simulink model "Simulink_model"  (R2024b)
settings: Solver=FixedStepAuto  StartTime=0.0  StopTime=10.0  FixedStep=1e-3  RelTol=1e-3
values from neighbouring files (symbols this model uses):
  A = [0 1; 0 -10]    [Script.m]
  B = [0; 120]    [Script.m]
  C = [1 0]    [Script.m]
  D = 0    [Script.m]
  Kd = (2*delta*omega_n+(-lambda3)-10)/(120)    [Script.m]
  Ki = (omega_n^2*(-lambda3))/(120)    (= 36)    [Script.m]
  Kp = (omega_n^2+2*delta*omega_n*(-lambda3))/(120)    [Script.m]
  Tl = 1/(8 * omega_n)    (= 0.0104166666667)    [Script.m]
settings Model: Creator=andre  LastModifiedBy=Enrico 2

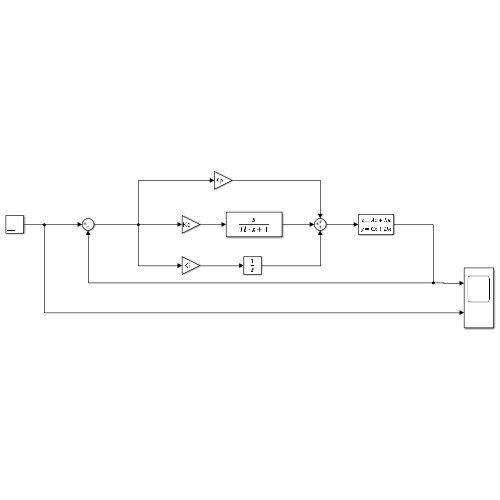
[thumbnail: Simulink's stored preview of the top-level diagram]
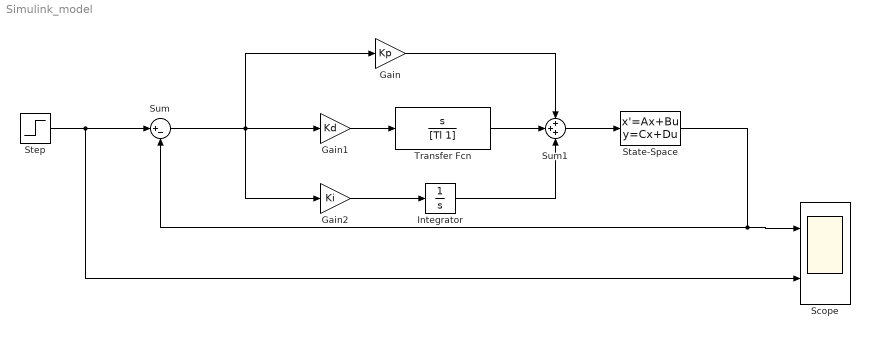
== system Simulink_model ==
  Gain : Gain  Gain=Kp
  Gain1 : Gain  Gain=Kd
  Gain2 : Gain  Gain=Ki
  Integrator : Integrator
  Scope : Scope  NumInputPorts=2
  State-Space : StateSpace  A=A  B=B  C=C  D=D  InitialCondition=0
  Step : Step  After=100  SampleTime=0
  Sum : Sum  Inputs=|+-
  Sum1 : Sum  Inputs=+++
  Transfer Fcn : TransferFcn  Numerator=[1 0]  Denominator=[Tl 1]
  wires:
  Step/1 -> Scope/2, Sum/1
  State-Space/1 -> Scope/1, Sum/2
  Gain/1 -> Sum1/1
  Gain1/1 -> Transfer Fcn/1
  Integrator/1 -> Sum1/3
  Gain2/1 -> Integrator/1
  Transfer Fcn/1 -> Sum1/2
  Sum1/1 -> State-Space/1
  Sum/1 -> Gain2/1, Gain1/1, Gain/1
